simulink model "D24_model"  (R2021a)
settings: Solver=VariableStepAuto  StartTime=0.0  StopTime=10.0  RelTol=1e-3
undefined symbols (not defined in the file or in its folder): Te
settings Model: Creator=djoroya  LastModifiedBy=djoroya

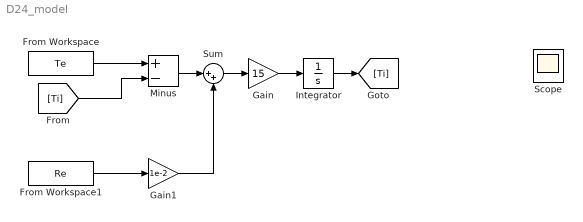
== system D24_model ==
  From Workspace : FromWorkspace  VariableName=Te
  From Workspace1 : FromWorkspace  VariableName=Re
  Gain : Gain  Gain=15
  Gain1 : Gain  Gain=1e-2
  Integrator : Integrator  InitialCondition=Te.signals.values(1)
  Minus : Sum  Inputs=+-
  Scope : Scope  NumInputPorts=2
  Sum : Sum  Inputs=|++
  wires:
  From Workspace/1 -> Minus/1
  Gain/1 -> Integrator/1
  Minus/1 -> Sum/1
  Sum/1 -> Gain/1
  From Workspace1/1 -> Gain1/1
  Gain1/1 -> Sum/2
  Integrator/1 -> [Ti]
  [Ti] -> Minus/2
